simulink model "onerobotcontroller"  (R2017a)
settings: Solver=VariableStepAuto  StartTime=0.0  StopTime=1000.0  RelTol=1e-3
undefined symbols (not defined in the file or in its folder): m, n
settings Model: Creator=admin  LastModifiedBy=admin

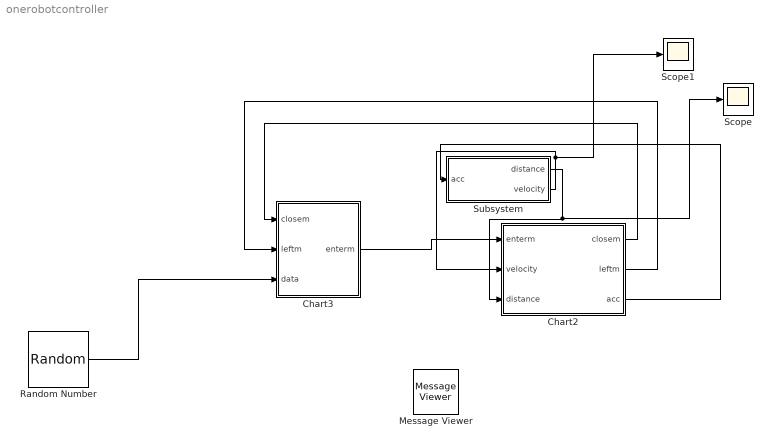
== system onerobotcontroller ==
  Chart2 : Stateflow chart  TreatAsAtomicUnit=on
  Chart3 : Stateflow chart  TreatAsAtomicUnit=on
  Message Viewer : MessageViewer  History=1000
  Random Number : RandomNumber  SampleTime=1
  Scope : Scope
  Scope1 : Scope
  Subsystem : Subsystem
  wires:
  Random Number/1 -> Chart3/3(data)
  Chart3/1(enterm) -> Chart2/1(enterm)
  Chart2/1(closem) -> Chart3/1(closem)
  Chart2/2(leftm) -> Chart3/2(leftm)
  Chart2/3(acc) -> Subsystem/1(acc)
  Subsystem/1(distance) -> Scope/1, Chart2/3(distance)
  Subsystem/2(velocity) -> Scope1/1, Chart2/2(velocity)

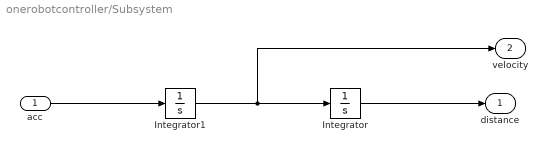
== system onerobotcontroller/Subsystem ==
  acc : Inport
  Integrator : Integrator  InitialCondition=50  WrapState=on  WrappedStateUpperValue=100  WrappedStateLowerValue=0
  Integrator1 : Integrator  InitialCondition=1
  distance : Outport
  velocity : Outport  Port=2
  wires:
  acc/1 -> Integrator1/1
  Integrator1/1 -> velocity/1, Integrator/1
  Integrator/1 -> distance/1

== stateflow chart onerobotcontroller/Chart2 ==
  state Move1
  state move3
    entry: acc = 0;
  state move2
  state decel_
    entry: acc=-0.01;
  state accel
    entry: acc = 0.01
  state stop
  move3 -> Move1 : [distance >= 1] {send(leftm)}
  (default) -> Move1
  Move1 -> move2 : [distance >= 70]
      | {send(closem)}
  move2 -> move3 [order 1] : enterm
  accel -> move3 : [velocity >= 1]
  move2 -> decel_ [order 2] : [distance >= 80]
  decel_ -> accel [order 2] : enterm
  decel_ -> stop [order 1] : [velocity <= 0 ]
      | {acc = 0}
  stop -> accel : enterm
  data: closem output double =1; leftm output double =1; enterm input double; acc output double =0; velocity input double; distance input double

== stateflow chart onerobotcontroller/Chart3 ==
  state robot_state1
  state robot_state2
    entry: x = 40*rand()+20
  state robot_state3
    entry:  send(enterm)
  robot_state3 -> robot_state1 : leftm
  (default) -> robot_state1
  robot_state1 -> robot_state2 : closem
  robot_state2 -> robot_state3 : after(x,sec)
  data: closem input double; leftm input double; data input; enterm output double =1; enter local; x local
